simulink model "test"  (Simulink 8.8)
settings: Solver=VariableStepAuto  StartTime=0.0  StopTime=50  RelTol=1e-3
settings Model: Creator=Wang  LastModifiedBy=Wang
settings DataIOCC: LimitDataPoints=off  SaveFormat=Dataset  SignalLoggingSaveFormat=Dataset
settings OptimizationCC: LifeSpan=auto
settings DebuggingCC: UnderspecifiedInitializationDetection=Simplified  MergeDetectMultiDrivingBlocksExec=error  FcnCallInpInsideContextMsg=error  StateNameClashWarn=none  SFUnexpectedBacktrackingDiag=error  SFNoUnconditionalDefaultTransitionDiag=error  SFExecutionAtInitializationDiag=warning
settings HardwareCC: ProdBitPerPointer=64  ProdBitPerSizeT=64  ProdBitPerPtrDiffT=64  ProdLargestAtomicFloat=Float  ProdIntDivRoundTo=Zero  ProdEndianess=LittleEndian  ProdWordSize=64  ProdHWDeviceType=Intel->x86-64 (Windows64)
settings ModelReferenceCC: PropagateSignalLabelsOutOfModel=on
settings GRTTargetCC: TargetLangStandard=C99 (ISO)  GeneratePreprocessorConditionals=Use local settings  CombineOutputUpdateFcns=on  GRTInterface=off
settings ConfigComp: CovMetricSettings=dwe  CovHtmlReporting=off  CovSaveCumulativeToWorkspaceVar=off  CovSaveSingleToWorkspaceVar=off  CovExternalEMLEnable=on

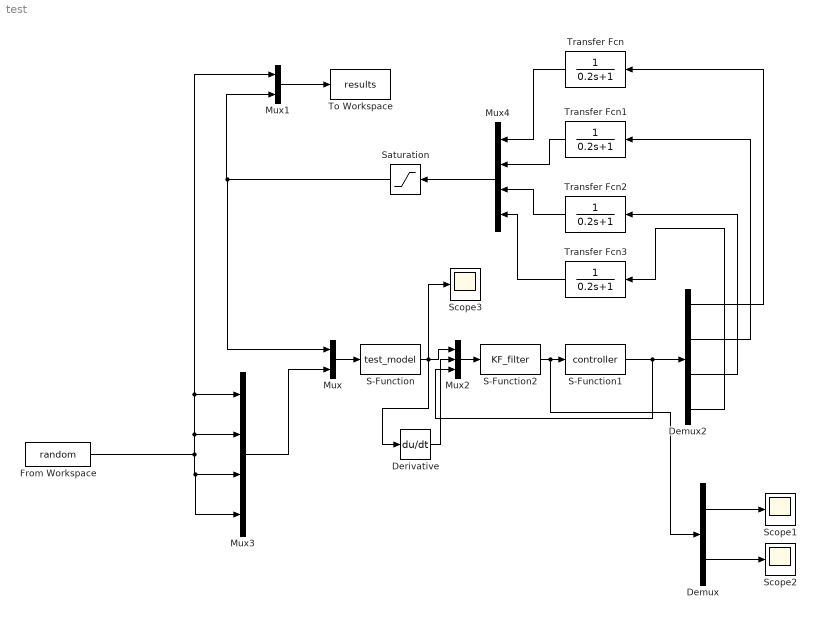
== system test ==
  Demux : Demux  Outputs=2
  Demux2 : Demux
  Derivative : Derivative
  From Workspace : FromWorkspace  VariableName=random  SampleTime=0
  Mux : Mux  Inputs=2
  Mux1 : Mux  Inputs=2
  Mux2 : Mux  Inputs=3
  Mux3 : Mux
  Mux4 : Mux
  S-Function : S-Function  FunctionName=test_model  SFunctionDeploymentMode=off  EnableBusSupport=off
  S-Function1 : S-Function  FunctionName=controller  SFunctionDeploymentMode=off  EnableBusSupport=off
  S-Function2 : S-Function  FunctionName=KF_filter  SFunctionDeploymentMode=off  EnableBusSupport=off
  Saturation : Saturate  UpperLimit=150  LowerLimit=-150
  Scope1 : Scope
  Scope2 : Scope
  Scope3 : Scope
  To Workspace : ToWorkspace  VariableName=results  SaveFormat=Timeseries  SampleTime=-1
  Transfer Fcn{,1..3} (4 alike) : TransferFcn  Denominator=[0.2 1]
  wires:
  Mux/1 -> S-Function/1
  From Workspace/1 -> Mux3/4, Mux3/3, Mux3/2, Mux3/1, Mux1/1
  Mux1/1 -> To Workspace/1
  Mux3/1 -> Mux/2
  Demux2/1 -> Transfer Fcn/1
  Transfer Fcn2/1 -> Mux4/3
  Transfer Fcn3/1 -> Mux4/4
  Transfer Fcn/1 -> Mux4/1
  Transfer Fcn1/1 -> Mux4/2
  S-Function1/1 -> Mux2/3, Demux2/1
  Demux2/2 -> Transfer Fcn1/1
  Demux2/3 -> Transfer Fcn2/1
  Demux2/4 -> Transfer Fcn3/1
  S-Function2/1 -> Demux/1, S-Function1/1
  Mux2/1 -> S-Function2/1
  S-Function/1 -> Derivative/1, Scope3/1, Mux2/1
  Demux/1 -> Scope1/1
  Demux/2 -> Scope2/1
  Derivative/1 -> Mux2/2
  Mux4/1 -> Saturation/1
  Saturation/1 -> Mux/1, Mux1/2
